simulink model "Slip_Hysteresis"  (R2023b)
settings: Solver=FixedStepDiscrete  StartTime=0.0  StopTime=10.0  RelTol=1e-3
model workspace (MAT data in the model file):
  slipActivateThreshold = Simulink.Parameter
  slipActivateThreshold.Value = 200
  slipActivateThreshold.DataType = 'uint16'
  slipActivateThreshold.Complexity = 'real'
  slipActivateThreshold.Dimensions = [1 1]
  slipDeactivateThreshold = Simulink.Parameter
  slipDeactivateThreshold.Value = 150
  slipDeactivateThreshold.DataType = 'uint16'
  slipDeactivateThreshold.Complexity = 'real'
  slipDeactivateThreshold.Dimensions = [1 1]
settings Model: ParameterArgumentNames=slipActivateThreshold,slipDeactivateThreshold  Creator=E8KUAVE  LastModifiedBy=E8KUAVE
settings OptimizationCC: DefaultParameterBehavior=Inlined  EnhancedBackFolding=on  PassReuseOutputArgsAs=Individual arguments  ZeroExternalMemoryAtStartup=off  ZeroInternalMemoryAtStartup=off  OptimizeBlockOrder=speed  DifferentSizesBufferReuse=on  OptimizationCustomize=off  EfficientTunableParamExpr=on
settings DebuggingCC: ParameterTunabilityLossMsg=error
settings HardwareCC: ProdBitPerPointer=32  ProdBitPerSizeT=32  ProdBitPerPtrDiffT=32  ProdLargestAtomicInteger=Long  ProdLargestAtomicFloat=Double  ProdWordSize=32  ProdHWDeviceType=ARM Compatible->ARM Cortex-M
settings SFSimCC: MATLABDynamicMemAlloc=off  SimTargetLang=C++
settings RTWCC: Description=Embedded Coder  SystemTargetFile=ert.tlc  GenCodeOnly=on  TemplateMakefile=ert_default_tmf  Toolchain=MinGW64 | gmake (64-bit Windows)  DataTypeReplacement=CDataTypesFixedWidth  TargetLang=C++
settings CodeAppCC: ForceParamTrailComments=on  IgnoreCustomStorageClasses=off  OperatorAnnotations=on  SimulinkDataObjDesc=on  SFDataObjDesc=on  InsertBlockDesc=on
settings ERTTargetCC: TargetLangStandard=C++11 (ISO)  GenerateSampleERTMain=on  CodeInterfacePackaging=C++ class  PurelyIntegerCode=on  SupportNonFinite=off  InlinedParameterPlacement=NonHierarchical  RootIOFormat=Structure reference  ERTCustomFileTemplate=example_file_process.tlc  MaxIdInt64=INT64_MAX  MinIdInt64=INT64_MIN  MaxIdUint64=UINT64_MAX  MaxIdInt32=INT32_MAX  MinIdInt32=INT32_MIN  MaxIdUint32=UINT32_MAX  MaxIdInt16=INT16_MAX  MinIdInt16=INT16_MIN  MaxIdUint16=UINT16_MAX  MaxIdInt8=INT8_MAX  MinIdInt8=INT8_MIN  MaxIdUint8=UINT8_MAX

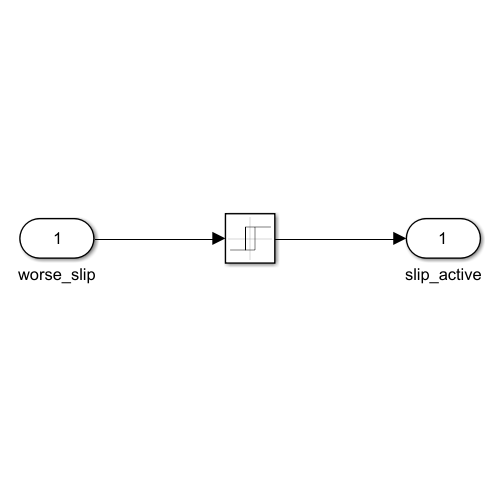
[thumbnail: Simulink's stored preview of the top-level diagram]
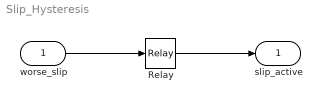
== system Slip_Hysteresis ==
  worse_slip : Inport  OutDataTypeStr=uint16
  Relay : Relay  OnSwitchValue=slipActivateThreshold  OffSwitchValue=slipDeactivateThreshold  OutDataTypeStr=boolean
  slip_active : Outport  OutDataTypeStr=boolean
  wires:
  worse_slip/1 -> Relay/1
  Relay/1 -> slip_active/1
